simulink model "Wind_Turbine_org"  (Simulink 10.0)
settings: Solver=ode23t  StartTime=0.0  StopTime=70  MaxStep=0.01  RelTol=1e-4  AbsTol=1e-4  EnableMultiTasking=on
PreLoadFcn:
  | warning off Simulink:Commands:LoadMdlParameterizedLink
PostLoadFcn:
  | warning off Simulink:blocks:MatchingGotoNotFound
  | warning off Simulink:blocks:MatchingFromNotFound
  | warning('off','Simulink:SL_OutputNotConnected');
  | warning off Simulink:Engine:SaveWithParameterizedLinks_Warning
  | warning off Simulink:Engine:SaveWithDisabledLinks_Warning
  | warning('off','Simulink:fixpoint:fxpParameterPrecisionLoss');
  | warning off Simulink:blocks:DTConversionUncessary
  | warning off ne_sli:simulator:input:FilteredInputs
  | warning off MATLAB:nearlySingularMatrix
  | 
  | warning off xPCTarget:modeloptions:StackIncrease
  | warning off xPCTarget:sampleTime:sampleTimeInvariance
  | warning off Simulink:blocks:TDelayFixedBuffer
  | 
  | Setup_WT_Configurations
StartFcn:
  | tic
StopFcn:
  | Elapsed_Sim_Time = toc;
  | disp(['Elapsed time is ' num2str(Elapsed_Sim_Time)]);
undefined symbols (not defined in the file): radps2rpm, sigbuilder_block, WT_Params, X, Y, Z
libraries: powerlib x6, sm_lib x6, Wind_Lib x4, Yaw_System_Lib x4, Generator_Lib x3, Pitch_System_Lib x3, Pitch_Controller_Lib x3, Main_Controller_Lib x2, Geartrain_Lib x2, Hub_Axis_Lib x2, Blades_Lib x1, nesl_utility x1
Description:
  | Copyright 2009-2017 The MathWorks, Inc. MathWorks, Inc.
settings Model: Creator=smiller  LastModifiedBy=bhisma  ExtModeTrigDuration=100
settings SolverCC: AutoScaleAbsTol=off  MaxConsecutiveMinStep=5
settings DataIOCC: SaveFinalState=on
settings OptimizationCC: BlockReduction=off  OptimizeBlockIOStorage=off  BufferReuse=off  GlobalBufferReuse=off  ExpressionFolding=off  ExpressionDepthLimit=2147483647  LocalBlockOutputs=off  OptimizeDataStoreBuffers=off  BusAssignmentInplaceUpdate=off
settings DebuggingCC: AlgebraicLoopMsg=error  ArtificialAlgebraicLoopMsg=none  Int32ToFloatConvMsg=none  UnnecessaryDatatypeConvMsg=warning  FcnCallInpInsideContextMsg=warning  AllowSymbolicDim=off  StateNameClashWarn=warning
settings HardwareCC: ProdIntDivRoundTo=Zero  ProdEndianess=LittleEndian  ProdLongLongMode=on  ProdHWDeviceType=Generic->32-bit x86 compatible  TargetBitPerLong=64  TargetBitPerPointer=64  TargetBitPerSizeT=64  TargetBitPerPtrDiffT=64  TargetLongLongMode=on  TargetIntDivRoundTo=Zero  TargetEndianess=LittleEndian  TargetWordSize=64  TargetHWDeviceType=MATLAB Host
settings SFSimCC: SimParseCustomCode=off
settings RTWCC: Description=Simulink Real-Time  SystemTargetFile=slrt.tlc  TemplateMakefile=slrt_default_tmf  RTWCompilerOptimization=on
settings TargetCC: CodeReplacementLibrary=XPC_BLAS  ParMdlRefBuildCompliant=on  ConcurrentExecutionCompliant=on  GeneratePreprocessorConditionals=Use local settings  MatFileLogging=on  PreserveStateflowLocalDataDimensions=off  MATLABClassNameForMDSCustomization=xpcAperiodicCustomization
settings CustomProperty: DataType=string
settings ConfigComp: CovExternalEMLEnable=off  CovSFcnEnable=off
settings SimscapeCC: ExplicitSolverDiagnosticOptions=none  SimscapeNormalizeSystem=off  SimscapeLogType=all  SimscapeLogName=simlog_Wind_Turbine  SimscapeLogLimitData=off
settings SimMechanicsCC: WarnOnRedundantConstraints=off  VisOnUpdateDiagram=on  VisDuringSimulation=on  FramesToBeSkipped=5  AnimationDelay=0  LastVizWinPosition=[16 233 560 424]  CamPosition=[-49.333;156.594;63.1057;]  CamTarget=[-1.98114;98.9678;-2.9194;]  CamUpVector=[0.335262;0.815674;-0.471461;]  CamHeight=16.8988  VisBackgroundColor=[0.678431;0.921569;1;]  DefaultBodyColor=[1;0;0;]
settings ConfigurationSet: Description=SimMechanics 2G
settings ExplorerConfigSet: InternalSimMechanicsExplorerSettings="<ExplorerConfiguration><canonicalview>default</canonicalview><TilePanel><TileInfo><Tiles Columns=\"2\" Count=\"3\" Rows=\"2\"><Column Left=\"2\" Weight=\"0.6616\"/><Column Left=\"1076\" Weight=\"0.3384\"/><Column Left=\"1628\"/><Row Top=\"2\" Weight=\"0.4995\"/><Row Top=\"507\" Weight=\"0.5005\"/><Row Top=\"1014\"/><Tile Height=\"1\" Width=\"1\" X=\"0\" Y=\"0\"/><Tile Height=\"1\" Width=\"1\" X=\"0\" Y=\"1\"/><Tile Height=\"2\" Width=\"1\" X=\"1\" Y=\"0\"/></Tiles></TileInfo><SceneInfo><SceneViewer><BGColor><R>0.80000001192092896</R><G>1</G><B>1</B></BGColor><Camera><Position><X>151.73049973570119</X><Y>118.34405364859263</Y><Z>134.40663706667596</Z></Position><Center><X>-10.795458452286731</X><Y>-8.3649508446642677</Y><Z>101.0263657071233</Z></Center><Up><X>-0.12932527544138767</X><Y>-0.094165770600414006</Y><Z>0.98712095549595125</Z></Up><Left>-10.158594940113018</Left><Right>10.158594940113018</Right><Bottom>-7.1278539082560997</Bottom><Top>7.1278539082560997</Top></Camera></SceneViewer><SceneViewer><BGColor><R>0.80000001192092896</R><G>1</G><B>1</B></BGColor><Camera><Position><X>3.5719318734898633</X><Y>-0.12848459366052295</Y><Z>225.51131574619058</Z></Position><Center><X>-2.4920494569662206</X><Y>-0.0648600322177105</Y><Z>66.260519833710546</Z></Center><Up><X>0.0026243051834802709</X><Y>-0.99999643177881292</Y><Z>-0.00049945164542893202</Z></Up><Left>-11.826399210226041</Left><Right>11.826399210226041</Right><Bottom>-5.4233487502515896</Bottom><Top>5.4233487502515896</Top></Camera></SceneViewer><SceneViewer><BGColor><R>0.80000001192092896</R><G>1</G><B>1</B></BGColor><Camera><Position><X>121.9852231624925</X><Y>91.296071561311123</Y><Z>95.392428744838412</Z></Position><Center><X>2.8343002263369788</X><Y>-1.5967499794196209</Y><Z>70.920706290818515</Z></Center><Up><X>-0.12932527544138767</X><Y>-0.094165770600414006</Y><Z>0.98712095549595125</Z></Up><Left>-36.268603134155278</Left><Right>36.268603134155278</Right><Bottom>-73.406224822998055</Bottom><Top>73.406224822998055</Top></Camera></SceneViewer></SceneInfo></TilePanel></ExplorerConfiguration>"

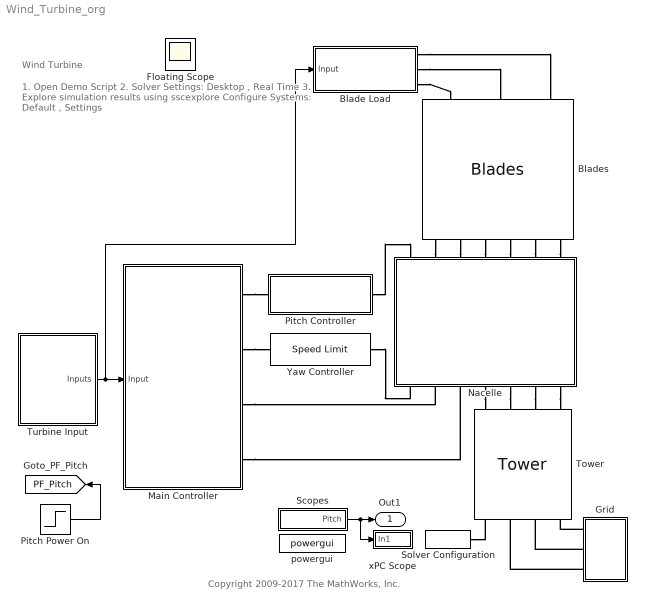
== system Wind_Turbine_org ==
  note: Copyright 2009-2017 The MathWorks, Inc.
  note: 1. Open Demo Script
      | 2. Solver Settings: Desktop , Real Time
      | 3. Explore simulation results using sscexplore
      |
      | Configure Systems: Default , Settings
  note: Wind Turbine
  Blade Load : Subsystem  VariantControlMode=Label  Variant=on  LabelModeActiveChoice=Lift_and_Drag
      settings: AttributesFormatString=%<ActiveVariant>
      mask Display:
      | blk = find_system(gcbh, 'SearchDepth', 1, 'Parent', gcb, 'VariantObject', get_param(gcb,'activevariant'));
      | eval(get_param(blk, 'MaskDisplay'));
  Blades : Blades_Lib/Blades  RequirementInfo={'other' 'wind_turbine_requirements.docx' '@overall_system' 'true' 'Blade Requirements' '' } %GIDa_b4b772d6_2a4e_4d26_8c7e_f4f3f2f69a80  SystemSampleTime=-1
  Grid : Subsystem  RequirementInfo={} %GIDa_31a9dfe5_a537_4323_9f13_a43c2adbc945
  Main Controller : Subsystem  VariantControlMode=Label  Variant=on  LabelModeActiveChoice=Wind_Input
      settings: AttributesFormatString=%<ActiveVariant>
      mask Display:
      | blk = find_system(gcbh, 'SearchDepth', 1, 'Parent', gcb, 'VariantObject', get_param(gcb,'activevariant'));
      | eval(get_param(blk, 'MaskDisplay'));
  Nacelle : Subsystem
      mask Display:
      | PiA_Char = get_param([bdroot '/Nacelle/Pitch System'],'ActiveVariant');
      | YaA_Char = get_param([bdroot '/Nacelle/Yaw System'],'ActiveVariant');
      | Hub_Char = get_param([bdroot '/Nacelle/Hub Axis'],'ActiveVariant');
      | Gea_Char = get_param([bdroot '/Nacelle/Geartrain'],'ActiveVariant');
      | Gen_Char = get_param([bdroot '/Nacelle/Generator'],'ActiveVariant');
      | 
      | if(length(YaA_Char)<7)
      |     YaA_Char = 'LockedL';
      | end
      | 
      | image_str = ['Pi' PiA_Char(1) 'Ya' upper(YaA_Char(7)) 'Hu' Hub_Char(1) 'Ge' Gea_Char(1) 'Gn' Gen_Char(1)];
      | try
      |     image(['Nacelle_' image_str '_IMAGE.jpg']);
      | catch
      |     image('Nacelle_IMAGE.jpg');
      | end
      | 
      | port_label('RConn',1,'YC');
      | port_label('RConn',2,'Br');
      | port_label('RConn',3,'G');
      | port_label('RConn',4,'T');
      | port_label('RConn',5,'GrVa');
      | port_label('RConn',6,'GrVb');
      | port_label('RConn',7,'GrVc');
      | port_label('LConn',1,'PC');
      | port_label('LConn',2,'B1');
      | port_label('LConn',3,'BPA1');
      | port_label('LConn',4,'B2');
      | port_label('LConn',5,'BPA2');
      | port_label('LConn',6,'B3');
      | port_label('LConn',7,'BPA3');
  Pitch Power On : Step  Time=20  Before=24  After=24  SampleTime=0
  Pitch Controller : Subsystem  VariantControlMode=Label  Variant=on  LabelModeActiveChoice=PI_on_AoA
      settings: AttributesFormatString=%<ActiveVariant>
      mask Display:
      | blk = find_system(gcbh, 'SearchDepth', 1, 'Parent', gcb, 'VariantObject', get_param(gcb,'activevariant'));
      | eval(get_param(blk, 'MaskDisplay'));
  Scopes : Subsystem
      mask Display: disp('Scopes');
  Solver Configuration : nesl_utility/Solver Configuration  PhysicalDomain=network_engine_domain  SubClassName=solver  LeftPortType=input  RightPortType=generic  Tones=[]  Harmonics=[]  SimulateNoise=off  Profile=off  UseLocalSampling=off  EnableSwitchedLinearOptims=on  FrequencyDomain=off  UseCCode=off  RelTol=0.001  AbsTol=1e-06  MinStep=1e-09  ToWorkspace=off  RevertToSquareIcSolve=off  NumHomotopyIterations=100  PhasorMode=off  PhasorModeNumHarmonics=1  DoDC=off  ResidualTolerance=1e-9  UseLocalSolver=off  LocalSolverChoice=NE_BACKWARD_EULER_ADVANCER  LocalSolverSampleTime=0.01  DoFixedCost=off  MaxNonlinIter=3  MaxModeIter=2  LinearAlgebra=Sparse  EquationFormulation=NE_TIME_EF  DelaysMemoryBudget=1024  AutomaticFiltering=on  FilteringTimeConstant=0.001  PartitionStorageMethod=AS_NEEDED  PartitionMemoryBudget=1024  PartitionMethod=FAST
  Tower : Tower/Tower  RequirementInfo={} %GIDa_4943b1c2_7ab1_472c_939d_e8be874b5a74  SystemSampleTime=-1
  Turbine Input : Subsystem  VariantControlMode=Label  Variant=on  LabelModeActiveChoice=Wind
      settings: AttributesFormatString=%<ActiveVariant>
      mask Display:
      | blk = find_system(gcbh, 'SearchDepth', 1, 'Parent', gcb, 'VariantObject', get_param(gcb,'activevariant'));
      | eval(get_param(blk, 'MaskDisplay'));
      | 
      | 
      | if strcmp(get_param(gcb,'activevariant'),'Wind')
      |     [gr_ind, l] = signalbuilder([gcb '/Wind/Wind Input'], 'activegroup');
      |     text(0.05,0.9,['Data ' num2str(gr_ind)]);
      | end
  Yaw Controller : Yaw_Controller_Lib/Speed Limit  SystemSampleTime=-1  OverrideUsingVariant=Speed_Limit
  powergui : powerlib/powergui  SimulationMode=Phasor  SampleTime=1e-1  frequency=60  Iterations=50  frequencyindice=60  Pbase=100e6  ErrMax=1e-4  UnitsV=kV  UnitsW=MW  buscounter=0  FunctionMessages=off  echomessages=off  EnableUseOfTLC=off  CurrentSourceSwitches=off  DisableSnubberDevices=off  DisableRonSwitches=off  DisableVfSwitches=off  DisplayEquations=off  AutomaticDiscreteSolvers=off  SolverType=Tustin  Interpol=off  ExternalGateDelay=off  methode=off  Ts=0  x0status=blocks  SPID=off  SwTol=0  HookPort=off  NonlinearTolerance=1e-4  nMaxIteration=100  ContinueOnMaxIteration=off  RestoreLinks=warning  ResistiveCurrentMeasurement=off  Frange=[0:2:500]  Ylog=off  Xlog=on  ShowGrid=off  save=off  variable=ZData  structure=0  ZoomFFT=on  StartTime=0.0  cycles=1  DisplayStyle=1  fundamental=60  FreqAxis=off  MaxFrequency=1000  frequencyindicesteady=1  RmsSteady=1  display=off
      settings: SourceProductName=Simscape Electrical
  xPC Scope : Subsystem
      mask Display: disp('SLRT')
  Out1 : Outport
  Floating Scope : Scope
  tag scope: PF_Pitch=global
  wires:
  Pitch Power On/1 -> [PF_Pitch]
  Turbine Input/1(Inputs) -> Main Controller/1(Input), Blade Load/1(Input)
  Scopes/1(Pitch) -> xPC Scope/1(In1), Out1/1
  connections:
  Blades/LConn1 -- Nacelle/LConn2
  Pitch Controller/RConn1 -- Nacelle/LConn1
  Main Controller/RConn1 -- Pitch Controller/LConn1
  Nacelle/RConn5 -- Tower/LConn2
  Nacelle/RConn4 -- Tower/LConn1
  Solver Configuration/RConn1 -- Tower/RConn1
  Blades/LConn5 -- Nacelle/LConn6
  Blades/LConn4 -- Nacelle/LConn5
  Blades/LConn3 -- Nacelle/LConn4
  Blades/LConn2 -- Nacelle/LConn3
  Blades/LConn6 -- Nacelle/LConn7
  Nacelle/RConn6 -- Tower/LConn3
  Nacelle/RConn7 -- Tower/LConn4
  Grid/RConn1 -- Tower/RConn4
  Grid/RConn2 -- Tower/RConn3
  Grid/RConn3 -- Tower/RConn2
  Main Controller/RConn2 -- Yaw Controller/LConn1
  Main Controller/RConn4 -- Nacelle/RConn3
  Main Controller/RConn3 -- Nacelle/RConn2
  Blade Load/RConn3 -- Blades/RConn1
  Blade Load/RConn2 -- Blades/RConn2
  Blade Load/RConn1 -- Blades/RConn3
  Yaw Controller/RConn1 -- Nacelle/RConn1

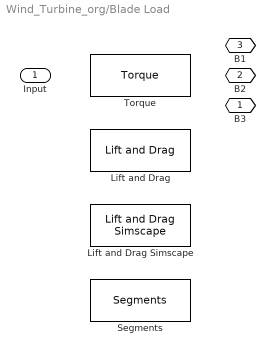
== system Wind_Turbine_org/Blade Load ==
  Input : Inport
  Lift and Drag : Wind_Lib/Lift and Drag  SystemSampleTime=-1  VariantControl=Lift_and_Drag
  Lift and Drag Simscape : Wind_Lib/Lift and Drag Simscape  SystemSampleTime=-1  VariantControl=Lift_and_Drag_Simscape
  Segments : Wind_Lib/Segments  SystemSampleTime=-1  VariantControl=Segments
  Torque : Wind_Lib/Torque  SystemSampleTime=-1  VariantControl=Torque
  B3 : PMIOPort  Side=Right
  B2 : PMIOPort  Port=2  Side=Right
  B1 : PMIOPort  Port=3  Side=Right

== system Wind_Turbine_org/Grid ==
  note: Copyright 2009-2017 The MathWorks, Inc.
  "1 km line " : powerlib/Elements/Three-Phase PI Section Line  LConnTagsString=a|b|c  RConnTagsString=A|B|C  Frequency=WT_Params.Grid.frequency  Resistances=[0.1153 0.413]  Inductances=[1.05e-3 3.32e-3]  Capacitances=[11.33e-009 5.01e-009]  Length=1
      settings: SourceProductName=Simscape Electrical
  Grid : powerlib/Electrical Sources/Three-Phase Programmable Voltage Source  PositiveSequence=[WT_Params.Grid.voltage 0 WT_Params.Grid.frequency]  VariationEntity=None  VariationType=Table of time-amplitude pairs  VariationTypeAlt=Step  VariationStep=-0.15  VariationRate=10  VariationMagnitude=0.3  VariationFrequency=2  VariationTiming=[5 5.5]  VariationPhaseA=off  Amplitudes="[1.0  0.5  1.0 ]"  TimeValues="[0  10  10.1]"  HarmonicGeneration=off  HarmonicA=[1 -0.1 0 1]  HarmonicB=[2 0.15 35 2]  Timing="[5  5.5]"  BusType=swing  Pref=0  Qref=0  Qmin=-inf  Qmax=inf
      settings: SourceProductName=Simscape Electrical
  Ground1 : powerlib/Elements/Ground  LConnTagsString=a
      settings: SourceProductName=Simscape Electrical
  Line Resistance : powerlib/Elements/Three-Phase Mutual Inductance Z1-Z0  LConnTagsString=a|b|c  RConnTagsString=A|B|C  PositiveSequence="[0.1  1.0/(2*pi*60)]*WT_Params.Grid.voltage^2/2500e6"  ZeroSequence="[0.3  3.0/(2*pi*60)]*WT_Params.Grid.voltage^2/2500e6"
      settings: SourceProductName=Simscape Electrical  SourceProductBaseCode=PS
  mGrid : powerlib/Measurements/Three-Phase V-I Measurement  VoltageMeasurement=phase-to-ground  SetLabelV=on  LabelV=VmGrid  Vpu=on  VpuLL=off  CurrentMeasurement=no  SetLabelI=on  LabelI=ImGrid  Ipu=off  Pbase=1.5e6/0.9  Vbase=25e3  OutputType=Magnitude  PhasorSimulation=on  PSBequivalent=0
      settings: SourceProductName=Simscape Electrical
  GNVc : PMIOPort  Side=Right
  GNVb : PMIOPort  Port=2  Side=Right
  GNVa : PMIOPort  Port=3  Side=Right
  connections:
  Line Resistance/RConn1 -- "1 km line "/LConn1
  "1 km line "/LConn2 -- Line Resistance/RConn2
  Line Resistance/RConn3 -- "1 km line "/LConn3
  Grid/LConn1 -- Ground1/LConn1
  Grid/RConn1 -- mGrid/LConn1
  mGrid/LConn2 -- Grid/RConn2
  Grid/RConn3 -- mGrid/LConn3
  mGrid/RConn1 -- Line Resistance/LConn1
  Line Resistance/LConn2 -- mGrid/RConn2
  mGrid/RConn3 -- Line Resistance/LConn3
  GNVa/RConn1 -- "1 km line "/RConn1
  GNVb/RConn1 -- "1 km line "/RConn2
  GNVc/RConn1 -- "1 km line "/RConn3

== system Wind_Turbine_org/Main Controller ==
  Input : Inport
  Direct Input : Main_Controller_Lib/Direct Input  SystemSampleTime=-1  VariantControl=Direct_Input
  Wind Input : Main_Controller_Lib/Wind Input  SystemSampleTime=-1  VariantControl=Wind_Input
  PC : PMIOPort  Tag=PMCPort  Side=Right
  YC : PMIOPort  Tag=PMCPort  Port=2  Side=Right
  Br : PMIOPort  Tag=PMCPort  Port=3  Side=Right
  G : PMIOPort  Tag=PMCPort  Port=4  Side=Right

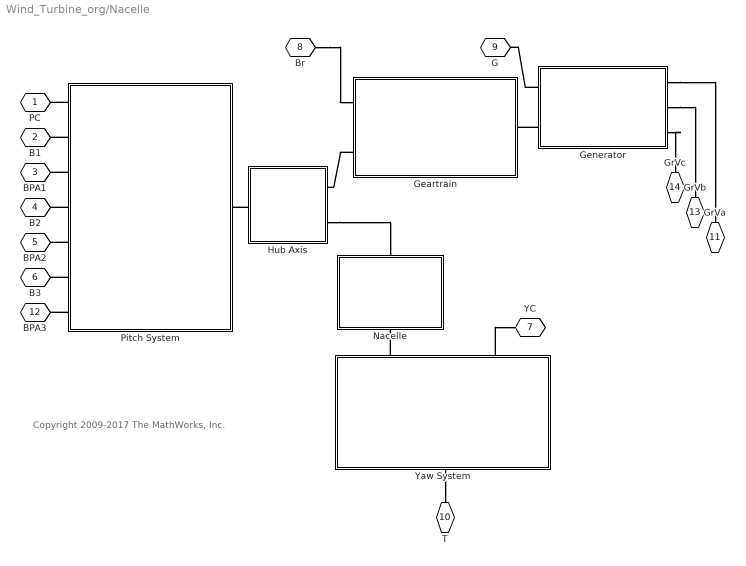
== system Wind_Turbine_org/Nacelle ==
  note: Copyright 2009-2017 The MathWorks, Inc.
  Geartrain : Subsystem  RequirementInfo={'other' 'Wind_Turbine_Requirements.docx' '@Simulink_requirement_item_4' 'true' 'Geartrain Requirements' '' } %GIDa_0de6bbf9_bd2a_4f23_951e_791819310b87  VariantControlMode=Label  Variant=on  LabelModeActiveChoice=Ideal
      settings: AttributesFormatString=%<ActiveVariant>
      mask Display:
      | blk = find_system(gcbh, 'SearchDepth', 1, 'Parent', gcb, 'VariantObject', get_param(gcb,'activevariant'));
      | eval(get_param(blk, 'MaskDisplay'));
  Generator : Subsystem  RequirementInfo={'other' 'Wind_Turbine_Requirements.docx' '@Simulink_requirement_item_5' 'true' 'Generator Requirements' '' } %GIDa_fc3d0265_e5fe_47b9_917a_323d12640d23  VariantControlMode=Label  Variant=on  LabelModeActiveChoice=Full
      settings: AttributesFormatString=%<ActiveVariant>
      mask Display:
      | blk = find_system(gcbh, 'SearchDepth', 1, 'Parent', gcb, 'VariantObject', get_param(gcb,'activevariant'));
      | eval(get_param(blk, 'MaskDisplay'));
  Hub Axis : Subsystem  Tag=CustomStyle  VariantControlMode=Label  Variant=on  LabelModeActiveChoice=Rotate
      settings: AttributesFormatString=%<ActiveVariant>
      mask Display:
      | blk = find_system(gcbh, 'SearchDepth', 1, 'Parent', gcb, 'VariantObject', get_param(gcb,'activevariant'));
      | eval(get_param(blk, 'MaskDisplay'));
  Nacelle : Subsystem
      mask Display:
      | image('Nacelle_Housing_IMAGE.jpg');
      | port_label('RConn',1,'N');
      | port_label('LConn',1,'YR');
  Pitch System : Subsystem  Tag=CustomStyle  VariantControlMode=Label  Variant=on  LabelModeActiveChoice=Ideal
      settings: AttributesFormatString=%<ActiveVariant>
      mask Display:
      | blk = find_system(gcbh, 'SearchDepth', 1, 'Parent', gcb, 'VariantObject', get_param(gcb,'activevariant'));
      | eval(get_param(blk, 'MaskDisplay'));
  Yaw System : Subsystem  Tag=CustomStyle  VariantControlMode=Label  Variant=on  LabelModeActiveChoice=Ideal_Actuator
      settings: AttributesFormatString=%<ActiveVariant>
      mask Display:
      | blk = find_system(gcbh, 'SearchDepth', 1, 'Parent', gcb, 'VariantObject', get_param(gcb,'activevariant'));
      | eval(get_param(blk, 'MaskDisplay'));
  PC : PMIOPort  Tag=PMCPort  Side=Left
  B1 : PMIOPort  Tag=PMCPort  Port=2  Side=Left
  BPA1 : PMIOPort  Tag=PMCPort  Port=3  Side=Left
  B2 : PMIOPort  Tag=PMCPort  Port=4  Side=Left
  BPA2 : PMIOPort  Tag=PMCPort  Port=5  Side=Left
  B3 : PMIOPort  Tag=PMCPort  Port=6  Side=Left
  YC : PMIOPort  Tag=PMCPort  Port=7  Side=Right
  Br : PMIOPort  Tag=PMCPort  Port=8  Side=Right
  G : PMIOPort  Tag=PMCPort  Port=9  Side=Right
  T : PMIOPort  Tag=PMCPort  Port=10  Side=Right
  GrVa : PMIOPort  Tag=PMCPort  Port=11  Side=Right
  BPA3 : PMIOPort  Tag=PMCPort  Port=12  Side=Left
  GrVb : PMIOPort  Tag=PMCPort  Port=13  Side=Right
  GrVc : PMIOPort  Tag=PMCPort  Port=14  Side=Right
  connections:
  Hub Axis/LConn1 -- Pitch System/RConn1
  Yaw System/RConn1 -- Nacelle/LConn1
  Yaw System/LConn1 -- T/RConn1
  Generator/RConn3 -- GrVc/RConn1
  Generator/RConn2 -- GrVb/RConn1
  Br/RConn1 -- Geartrain/LConn1
  Pitch System/LConn7 -- BPA3/RConn1
  Pitch System/LConn5 -- BPA2/RConn1
  Pitch System/LConn3 -- BPA1/RConn1
  Pitch System/LConn6 -- B3/RConn1
  Generator/LConn2 -- Geartrain/RConn1
  Generator/LConn1 -- G/RConn1
  Generator/RConn1 -- GrVa/RConn1
  Pitch System/LConn1 -- PC/RConn1
  Pitch System/LConn4 -- B2/RConn1
  Pitch System/LConn2 -- B1/RConn1
  Hub Axis/RConn2 -- Nacelle/RConn1
  Yaw System/RConn2 -- YC/RConn1
  Geartrain/LConn2 -- Hub Axis/RConn1

== system Wind_Turbine_org/Pitch Controller ==
  Inner Loop : Pitch_Controller_Lib/Inner Loop  SystemSampleTime=-1  VariantControl=Inner_Loop
  PI on AoA : Pitch_Controller_Lib/PI on AoA  SystemSampleTime=-1  VariantControl=PI_on_AoA
  PI on AoA Code : Pitch_Controller_Lib/PI on AoA Code  SystemSampleTime=-1  VariantControl=PI_on_AoA_Code
  P : PMIOPort  Tag=PMCPort  Side=Right
  M : PMIOPort  Tag=PMCPort  Port=2  Side=Left

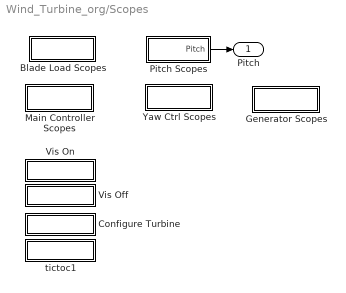
== system Wind_Turbine_org/Scopes ==
  Blade Load Scopes : Subsystem  AncestorBlock=Wind_Lib/Blade Load Scopes
  Configure Turbine : Subsystem
      mask Display: disp('Configs');
  Generator Scopes : Subsystem  AncestorBlock=Generator_Lib/Generator Scopes
  Main Controller Scopes : Subsystem  AncestorBlock=Main_Controller_Lib/Main Controller Scopes
  Pitch Scopes : Subsystem  AncestorBlock=Pitch_Controller_Lib/Pitch Scopes
  Vis Off : Subsystem
      settings: OpenFcn=set_param(bdroot,'SimMechanicsOpenEditorOnUpdate','off');
      mask Display: disp('Vis Off')
  Vis On : Subsystem
      settings: OpenFcn=set_param(bdroot,'SimMechanicsOpenEditorOnUpdate','on');
      mask Display: disp('Vis On')
  Yaw Ctrl Scopes : Subsystem  AncestorBlock=Yaw_Controller_Lib/Yaw Ctrl Scopes
  tictoc1 : Subsystem
      settings: OpenFcn=open('Wind_Turbine_Demo_Script.html')
      mask Display: disp('Script')
  Pitch : Outport
  wires:
  Pitch Scopes/1(Pitch) -> Pitch/1

== system Wind_Turbine_org/Turbine Input ==
  Commands : Subsystem  VariantControl=Commands
      mask Display:
      | image(imread('Turbine_Input_Commands_IMAGE.jpg'));
      | port_label('output',1,'Inputs');
  Wind : Subsystem  VariantControl=Wind
      mask Display:
      | image('Turbine_Input_Wind_IMAGE.jpg');
      | port_label('output',1,'Inputs');
  Inputs : Outport

== system Wind_Turbine_org/xPC Scope ==
  In1 : Inport
  "Scope (SLRT) " : slrtlib/Displays and Logging/Scope   scopeno=1  scopetype=Target  autostart=on  viewmode=Graphical redraw  formatstr='%15.6f'  grid=on  ylimits=[-5 70]  nosamples=200  noprepostsamples=0  interleave=1  triggermode=FreeRun  triggersignal=1  trigsignalfromport=off  triggerlevel=0.0  triggerslope=Either  triggerscope=1  triggersample=0  filename=data.dat  mode=Lazy  writesize=512  autorestart=off  dynamicfilemode=off  maxwritefilesize=512*1024^2
  wires:
  In1/1 -> "Scope (SLRT) "/1

== system Wind_Turbine_org/Nacelle/Geartrain ==
  Empty : Geartrain_Lib/Empty  SystemSampleTime=-1  VariantControl=Empty
  Ideal : Geartrain_Lib/Ideal  SystemSampleTime=-1  VariantControl=Ideal
  BC : PMIOPort  Tag=PMCPort  Side=Left
  R : PMIOPort  Tag=PMCPort  Port=2  Side=Left
  GN : PMIOPort  Tag=PMCPort  Port=3  Side=Right

== system Wind_Turbine_org/Nacelle/Generator ==
  Full : Generator_Lib/Full  SystemSampleTime=-1  VariantControl=Full
  Simple : Generator_Lib/Simple  SystemSampleTime=-1  VariantControl=Simple
  M : PMIOPort  Tag=PMCPort  Side=Left
  G : PMIOPort  Port=2  Side=Left
  GrVa : PMIOPort  Port=3  Side=Right
  GrVb : PMIOPort  Port=4  Side=Right
  GrVc : PMIOPort  Port=5  Side=Right

== system Wind_Turbine_org/Nacelle/Hub Axis ==
  Locked : Hub_Axis_Lib/Locked  SystemSampleTime=-1  VariantControl=Locked
  Rotate : Hub_Axis_Lib/Rotate  SystemSampleTime=-1  VariantControl=Rotate
  G : PMIOPort  Side=Right
  R : PMIOPort  Port=2  Side=Left
  N : PMIOPort  Port=3  Side=Right

== system Wind_Turbine_org/Nacelle/Nacelle ==
  Geometry : sm_lib/Body Elements/Extruded Solid  GraphicAmbientColor=[0.15 0.15 0.15 1.0]  BasedOnType=Density  CenterOfMass=[0 0 0]  CenterOfMassUnits=m  GraphicDiffuseColor=[0.8 0.8 0.8]  ExtrusionCrossSection=WT_Params.Nacelle.Geometry.profile  ExtrusionCrossSectionUnits=m  Density=1000  DensityUnits=kg/(m^3)  DoExposeReferenceFrame=on  GraphicEmissiveColor=[0.0 0.0 0.0 1.0]  ExportEntireGeometry=off  ExtrusionLength=WT_Params.Nacelle.length  ExtrusionLengthUnits=m  ExtrusionType=General  SerializedFrames=<Frames/>  MarkerShape=Sphere  MarkerSize=10  GraphicType=FromGeometry  InertiaType=PointMass  Mass=0.1  MassUnits=kg  MomentsOfInertia=[1 1 1]  MomentsOfInertiaUnits=kg*m^2  PolygonNumSides=3  GraphicOpacity=1.0  PolygonOuterRadius=1  PolygonOuterRadiusUnits=m  ProductsOfInertia=[0 0 0]  ProductsOfInertiaUnits=kg*m^2  GraphicShininess=75  GraphicSpecularColor=[0.5 0.5 0.5 1.0]  GraphicVisPropType=SimpleVisualProperties
      settings: SourceProductName=Simscape Multibody
  Inertia : sm_lib/Body Elements/Spherical Solid  GraphicAmbientColor=[0.15 0.15 0.15 1.0]  BasedOnType=Density  CenterOfMass=[0 0 0]  CenterOfMassUnits=m  GraphicDiffuseColor=[0.8 0.8 0.8]  Density=1000  DensityUnits=kg/(m^3)  DoExposeReferenceFrame=on  GraphicEmissiveColor=[0.0 0.0 0.0 1.0]  ExportEntireGeometry=off  SerializedExposedGeometries=<ExposedGeometries/>  SerializedFrames=<Frames/>  MarkerShape=Sphere  MarkerSize=10  GraphicType=FromGeometry  InertiaType=Custom  Mass=WT_Params.Nacelle.mass  MassUnits=kg  MomentsOfInertia=[WT_Params.Nacelle.inertia(1,1) WT_Params.Nacelle.inertia(3,3) WT_Params.Nacelle.inertia(2,2)]  MomentsOfInertiaUnits=kg*m^2  GraphicOpacity=1.0  ProductsOfInertia=[0 0 0]  ProductsOfInertiaUnits=kg*m^2  GraphicShininess=75  GraphicSpecularColor=[0.5 0.5 0.5 1.0]  SphereRadius=0.1  SphereRadiusUnits=m  GraphicVisPropType=SimpleVisualProperties
      settings: SourceProductName=Simscape Multibody
  Transform Extrusion : sm_lib/Frames and Transforms/Rigid Transform  TranslationMethod=Cartesian  TranslationStandardOffset=1  TranslationLengthUnit=m  TranslationStandardAxis=+Z  TranslationCartesianOffset=[0 0 0]  TranslationROffset=0  TranslationROffsetUnits=m  TranslationZOffset=0  TranslationZOffsetUnits=m  TranslationThetaOffset=0  TranslationThetaOffsetUnits=deg  RotationMethod=StandardAxis  RotationAngleUnits=deg  RotationStandardAxis=+Y  RotationAngle=90  RotationArbitraryAxis=[0 0 1]  FollAlignAxisA=+X  BaseAlignAxisA=+Y  FollAlignAxisB=+Y  BaseAlignAxisB=+Z  RotationSequenceAxes=FollowerAxes  RotationSequence=XYX  RotationSequenceAngles=[0 0 0]  RotationSequenceAnglesUnits=deg  RotationMatrix=[1 0 0; 0 1 0; 0 0 1]
  Transform Hub Center : sm_lib/Frames and Transforms/Rigid Transform  TranslationMethod=StandardAxis  TranslationStandardOffset=WT_Params.Nacelle.length/2  TranslationLengthUnit=m  TranslationStandardAxis=+X  TranslationCartesianOffset=[0 0 0]  TranslationROffset=0  TranslationROffsetUnits=m  TranslationZOffset=0  TranslationZOffsetUnits=m  TranslationThetaOffset=0  TranslationThetaOffsetUnits=deg  RotationMethod=StandardAxis  RotationAngleUnits=deg  RotationStandardAxis=+Y  RotationAngle=90  RotationArbitraryAxis=[0 0 1]  FollAlignAxisA=+X  BaseAlignAxisA=+Y  FollAlignAxisB=+Y  BaseAlignAxisB=+Z  RotationSequenceAxes=FollowerAxes  RotationSequence=XYX  RotationSequenceAngles=[0 0 0]  RotationSequenceAnglesUnits=deg  RotationMatrix=[1 0 0; 0 1 0; 0 0 1]
  Transform Nacelle CG : sm_lib/Frames and Transforms/Rigid Transform  TranslationMethod=Cartesian  TranslationStandardOffset=1  TranslationLengthUnit=m  TranslationStandardAxis=+Z  TranslationCartesianOffset=[-WT_Params.Nacelle.Yaw_Ctr_Offset.x+WT_Params.Nacelle.CG_Offset.x 0 WT_Params.Nacelle.Yaw_Ctr_Offset.y]  TranslationROffset=0  TranslationROffsetUnits=m  TranslationZOffset=0  TranslationZOffsetUnits=m  TranslationThetaOffset=0  TranslationThetaOffsetUnits=deg  RotationMethod=None  RotationAngleUnits=deg  RotationStandardAxis=+Z  RotationAngle=0  RotationArbitraryAxis=[0 0 1]  FollAlignAxisA=+X  BaseAlignAxisA=+Y  FollAlignAxisB=+Y  BaseAlignAxisB=+Z  RotationSequenceAxes=FollowerAxes  RotationSequence=XYX  RotationSequenceAngles=[0 0 0]  RotationSequenceAnglesUnits=deg  RotationMatrix=[1 0 0; 0 1 0; 0 0 1]
  Transform Nacelle Ctr : sm_lib/Frames and Transforms/Rigid Transform  TranslationMethod=Cartesian  TranslationStandardOffset=1  TranslationLengthUnit=m  TranslationStandardAxis=+Z  TranslationCartesianOffset=[-WT_Params.Nacelle.length/2+3 0 WT_Params.Nacelle.Yaw_Ctr_Offset.y]  TranslationROffset=0  TranslationROffsetUnits=m  TranslationZOffset=0  TranslationZOffsetUnits=m  TranslationThetaOffset=0  TranslationThetaOffsetUnits=deg  RotationMethod=None  RotationAngleUnits=deg  RotationStandardAxis=+Z  RotationAngle=0  RotationArbitraryAxis=[0 0 1]  FollAlignAxisA=+X  BaseAlignAxisA=+Y  FollAlignAxisB=+Y  BaseAlignAxisB=+Z  RotationSequenceAxes=FollowerAxes  RotationSequence=XYX  RotationSequenceAngles=[0 0 0]  RotationSequenceAnglesUnits=deg  RotationMatrix=[1 0 0; 0 1 0; 0 0 1]
  N : PMIOPort  Side=Right
  YR : PMIOPort  Port=2  Side=Left
  connections:
  Transform Nacelle Ctr/LConn1 -- YR/RConn1 -- Transform Nacelle CG/LConn1
  Transform Nacelle Ctr/RConn1 -- Transform Extrusion/LConn1 -- Transform Hub Center/LConn1
  Transform Hub Center/RConn1 -- N/RConn1
  Inertia/RConn1 -- Transform Nacelle CG/RConn1
  Transform Extrusion/RConn1 -- Geometry/RConn1

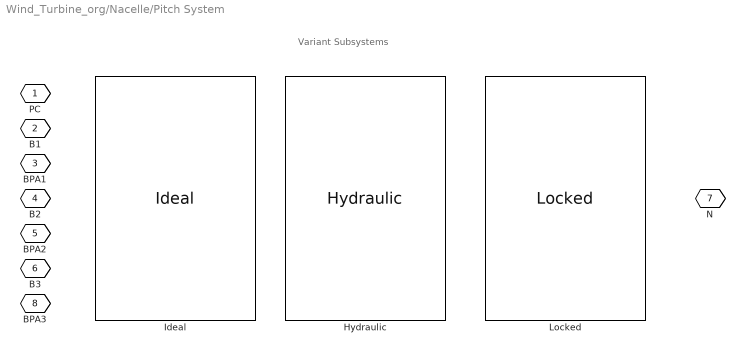
== system Wind_Turbine_org/Nacelle/Pitch System ==
  note: Variant Subsystems
  Hydraulic : Pitch_System_Lib/Hydraulic  SystemSampleTime=-1  VariantControl=Hydraulic
  Ideal : Pitch_System_Lib/Ideal  SystemSampleTime=-1  VariantControl=Ideal
  Locked : Pitch_System_Lib/Locked  SystemSampleTime=-1  VariantControl=Locked
  PC : PMIOPort  Tag=PMCPort  Side=Left
  B1 : PMIOPort  Tag=PMCPort  Port=2  Side=Left
  BPA1 : PMIOPort  Tag=PMCPort  Port=3  Side=Left
  B2 : PMIOPort  Tag=PMCPort  Port=4  Side=Left
  BPA2 : PMIOPort  Tag=PMCPort  Port=5  Side=Left
  B3 : PMIOPort  Tag=PMCPort  Port=6  Side=Left
  N : PMIOPort  Tag=PMCPort  Port=7  Side=Right
  BPA3 : PMIOPort  Tag=PMCPort  Port=8  Side=Left

== system Wind_Turbine_org/Nacelle/Yaw System ==
  Ideal Actuator : Yaw_System_Lib/Ideal Actuator  SystemSampleTime=-1  VariantControl=Ideal_Actuator
  Ideal Motor : Yaw_System_Lib/Ideal Motor  SystemSampleTime=-1  VariantControl=Ideal_Motor
  Locked : Yaw_System_Lib/Locked  SystemSampleTime=-1  VariantControl=Locked
  Servomotor : Yaw_System_Lib/Servomotor  SystemSampleTime=-1  VariantControl=Servomotor
  N : PMIOPort  Side=Right
  T : PMIOPort  Port=2  Side=Left
  YC : PMIOPort  Port=3  Side=Right

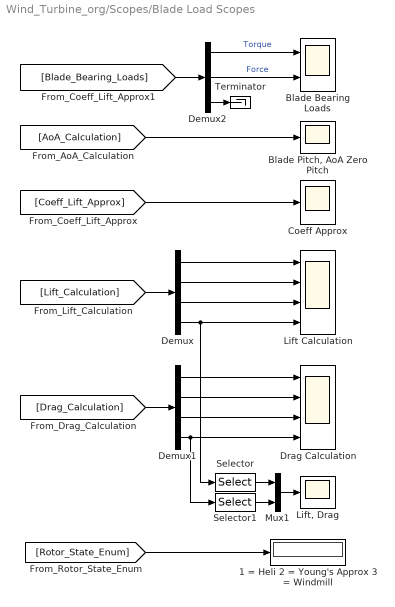
== system Wind_Turbine_org/Scopes/Blade Load Scopes ==
  1 = Heli 2 = Young's Approx 3 = Windmill : Display
  Blade Bearing Loads : Scope  NumInputPorts=2
  "Blade Pitch, AoA Zero Pitch" : Scope
  Coeff Approx : Scope
  Demux : Demux  Outputs=[1 3 3 3]
  Demux1 : Demux  Outputs=[1 3 3 3]
  Demux2 : Demux  Outputs=[3 3 12]
  Drag Calculation : Scope  NumInputPorts=4
  Lift Calculation : Scope  NumInputPorts=4
  "Lift, Drag" : Scope
  Mux1 : Mux  Inputs=2
  Selector : Selector  InputPortWidth=3  IndexOptions=Index vector (dialog)  Indices=[1]  OutputSizes=1
  Selector1 : Selector  InputPortWidth=3  IndexOptions=Index vector (dialog)  Indices=[1 3]  OutputSizes=1
  Terminator : Terminator
  wires:
  Demux2/3 -> Terminator/1
  [Rotor_State_Enum] -> 1 = Heli 2 = Young's Approx 3 = Windmill/1
  Demux1/4 -> Drag Calculation/4, Selector1/1
  Demux1/3 -> Drag Calculation/3
  Demux1/2 -> Drag Calculation/2
  Demux1/1 -> Drag Calculation/1
  [Drag_Calculation] -> Demux1/1
  [Coeff_Lift_Approx] -> Coeff Approx/1
  Demux/4 -> Lift Calculation/4, Selector/1
  Demux/3 -> Lift Calculation/3
  Demux/2 -> Lift Calculation/2
  Demux/1 -> Lift Calculation/1
  [Lift_Calculation] -> Demux/1
  Mux1/1 -> "Lift, Drag"/1
  [AoA_Calculation] -> "Blade Pitch, AoA Zero Pitch"/1
  Selector/1 -> Mux1/1
  Selector1/1 -> Mux1/2
  [Blade_Bearing_Loads] -> Demux2/1
  Demux2/1 -> Blade Bearing Loads/1  "Torque"
  Demux2/2 -> Blade Bearing Loads/2  "Force"

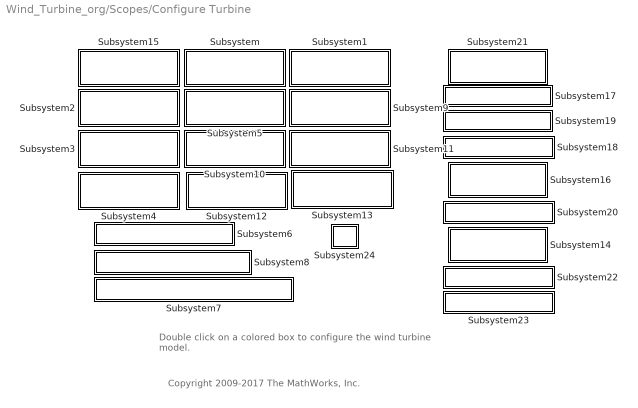
== system Wind_Turbine_org/Scopes/Configure Turbine ==
  note: Copyright 2009-2017 The MathWorks, Inc.
  note: Double click on a colored box
      | to configure the wind turbine model.
  Subsystem : Subsystem
      settings: OpenFcn=Select_Turbine_Systems('I_Pitch Test', WT_Configs)
      mask Display: disp('Ideal\nPitch')
  Subsystem1 : Subsystem
      settings: OpenFcn=Select_Turbine_Systems('H_Pitch Test', WT_Configs)
      mask Display: disp('Hydraulic\nPitch')
  Subsystem10 : Subsystem
      settings: OpenFcn=Select_Turbine_Systems('I_Pitch IM_Yaw Test', WT_Configs)
      mask Display: disp('Ideal Pitch\nIdeal Motor Yaw')
  Subsystem11 : Subsystem
      settings: OpenFcn=Select_Turbine_Systems('H_Pitch IM_Yaw Test', WT_Configs)
      mask Display: disp('Hydraulic Pitch\nIdeal Motor Yaw')
  Subsystem12 : Subsystem
      settings: OpenFcn=Select_Turbine_Systems('I_Pitch S_Yaw Test', WT_Configs)
      mask Display: disp('Ideal Pitch\nServomotor Yaw')
  Subsystem13 : Subsystem
      settings: OpenFcn=Select_Turbine_Systems('H_Pitch S_Yaw Test', WT_Configs)
      mask Display: disp('Hydraulic Pitch\nServomotor Yaw')
  Subsystem14 : Subsystem
      settings: OpenFcn=Compare_Yaw_Actuators;
      mask Display: disp('Compare Yaw\nActuators')
  Subsystem15 : Subsystem
      mask Display: disp('TESTS')
  Subsystem16 : Subsystem
      settings: OpenFcn=Compare_Pitch_Actuators;
      mask Display: disp('Compare Pitch\nActuators')
  Subsystem17 : Subsystem
      settings: OpenFcn=Pitch_Actuation_Linkage
      mask Display: disp('Pitch Linkage')
  Subsystem18 : Subsystem
      settings: OpenFcn=Pitch_Actuation_Hydraulic_Testrig
      mask Display: disp('Hydr. Pitch Testrig')
  Subsystem19 : Subsystem
      settings: OpenFcn=Pitch_Control_Ideal_Testrig
      mask Display: disp('Ideal Pitch Testrig')
  Subsystem2 : Subsystem
      settings: OpenFcn=Select_Turbine_Systems('IA_Yaw Test', WT_Configs)
      mask Display: disp('Ideal Actuator\nYaw')
  Subsystem20 : Subsystem
      settings: OpenFcn=Yaw_Actuation_Testrig
      mask Display: disp('Yaw Testrig')
  Subsystem21 : Subsystem
      mask Display: disp('DEVELOP')
  Subsystem22 : Subsystem
      settings: OpenFcn=Generator_Testrig
      mask Display: disp('Generator Testrig')
  Subsystem23 : Subsystem
      settings: OpenFcn=Turbine_State_Machine_Testrig
      mask Display: disp('Supervisory Ctrl')
  Subsystem24 : Subsystem
      settings: OpenFcn=Select_Turbine_Systems('H_Pitch S_Yaw Ge Gn Lift_Drag', WT_Configs)
      mask Display: disp('C')
  Subsystem3 : Subsystem
      settings: OpenFcn=Select_Turbine_Systems('IM_Yaw Test', WT_Configs)
      mask Display: disp('Ideal Motor\nYaw')
  Subsystem4 : Subsystem
      settings: OpenFcn=Select_Turbine_Systems('S_Yaw Test', WT_Configs)
      mask Display: disp('Servomotor\nYaw')
  Subsystem5 : Subsystem
      settings: OpenFcn=Select_Turbine_Systems('I_Pitch IA_Yaw Test', WT_Configs)
      mask Display: disp('Ideal Pitch\nIdeal Act. Yaw')
  Subsystem6 : Subsystem
      settings: OpenFcn=Select_Turbine_Systems('I_Pitch IA_Yaw Lift_Drag', WT_Configs)
      mask Display: disp('I Pitch IA Yaw Lift Drag')
  Subsystem7 : Subsystem
      settings: OpenFcn=Select_Turbine_Systems('I_Pitch IA_Yaw Ge Gn Lift_Drag', WT_Configs)
      mask Display: disp('I_Pitch IA_Yaw Ge Gn Lift_Drag')
  Subsystem8 : Subsystem
      settings: OpenFcn=Select_Turbine_Systems('I_Pitch IA_Yaw Ge Lift_Drag', WT_Configs)
      mask Display: disp('I Pitch IA Yaw Ge Lift Drag')
  Subsystem9 : Subsystem
      settings: OpenFcn=Select_Turbine_Systems('H_Pitch IA_Yaw Test', WT_Configs)
      mask Display: disp('Hydraulic Pitch\nIdeal Act. Yaw')

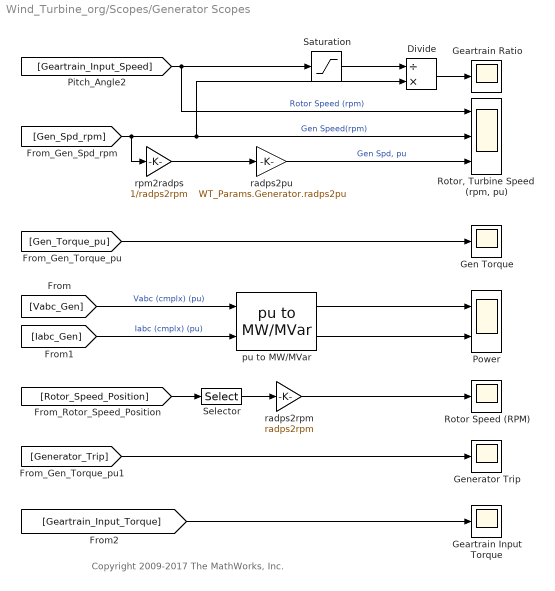
== system Wind_Turbine_org/Scopes/Generator Scopes ==
  note: Copyright 2009-2017 The MathWorks, Inc.
  Divide : Product  Inputs=/*
  Geartrain Input Torque : Scope
  Geartrain Ratio : Scope
  Gen Torque : Scope
  Generator Trip : Scope
  Power : Scope  NumInputPorts=2
  Rotor Speed (RPM) : Scope
  "Rotor, Turbine Speed  (rpm, pu)" : Scope  NumInputPorts=3
  Saturation : Saturate  UpperLimit=inf  LowerLimit=eps
  Selector : Selector  InputPortWidth=2  IndexOptions=Index vector (dialog)  Indices=[2]  OutputSizes=1
  pu to MW/MVar : Generator_Lib/Generator Scopes/pu to MW//MVar
  radps2pu : Gain  Gain=WT_Params.Generator.radps2pu
  radps2rpm : Gain  Gain=radps2rpm
  rpm2radps : Gain  Gain=1/radps2rpm
  wires:
  [Generator_Trip] -> Generator Trip/1
  pu to MW/MVar/2 -> Power/2
  pu to MW/MVar/1 -> Power/1
  [Gen_Torque_pu] -> Gen Torque/1
  [Iabc_Gen] -> pu to MW/MVar/2  "Iabc (cmplx) (pu)"
  [Vabc_Gen] -> pu to MW/MVar/1  "Vabc (cmplx) (pu)"
  [Geartrain_Input_Speed] -> "Rotor, Turbine Speed  (rpm, pu)"/1, Saturation/1  "Rotor Speed (rpm)"
  radps2pu/1 -> "Rotor, Turbine Speed  (rpm, pu)"/3  "Gen Spd, pu"
  rpm2radps/1 -> radps2pu/1
  Divide/1 -> Geartrain Ratio/1
  [Gen_Spd_rpm] -> "Rotor, Turbine Speed  (rpm, pu)"/2, Divide/2, rpm2radps/1  "Gen Speed(rpm)"
  [Rotor_Speed_Position] -> Selector/1
  Selector/1 -> radps2rpm/1
  radps2rpm/1 -> Rotor Speed (RPM)/1
  Saturation/1 -> Divide/1
  [Geartrain_Input_Torque] -> Geartrain Input Torque/1

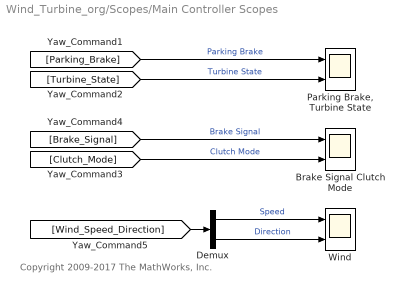
== system Wind_Turbine_org/Scopes/Main Controller Scopes ==
  note: Copyright 2009-2017 The MathWorks, Inc.
  Brake Signal Clutch Mode : Scope  NumInputPorts=2
  Demux : Demux  Outputs=2
  "Parking Brake, Turbine State" : Scope  NumInputPorts=2
  Wind : Scope  NumInputPorts=2
  wires:
  [Parking_Brake] -> "Parking Brake, Turbine State"/1  "Parking Brake"
  [Turbine_State] -> "Parking Brake, Turbine State"/2  "Turbine State"
  [Brake_Signal] -> Brake Signal Clutch Mode/1  "Brake Signal"
  [Clutch_Mode] -> Brake Signal Clutch Mode/2  "Clutch Mode"
  [Wind_Speed_Direction] -> Demux/1
  Demux/1 -> Wind/1  "Speed"
  Demux/2 -> Wind/2  "Direction"

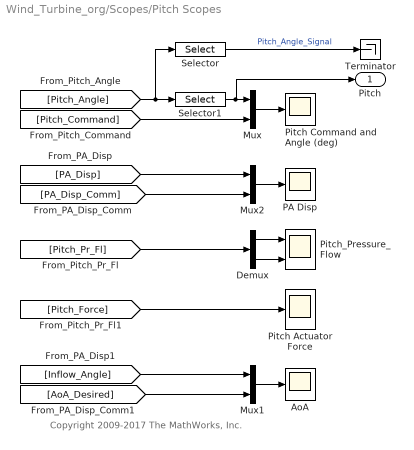
== system Wind_Turbine_org/Scopes/Pitch Scopes ==
  note: Copyright 2009-2017 The MathWorks, Inc.
  AoA : Scope
  Demux : Demux  Outputs=[2 1]
  Mux : Mux  Inputs=2
  Mux1 : Mux  Inputs=2
  Mux2 : Mux  Inputs=2
  PA Disp : Scope
  Pitch Actuator Force : Scope
  Pitch Command and Angle (deg) : Scope
  Pitch_Pressure_Flow : Scope  NumInputPorts=2
  Selector : Selector  InputPortWidth=3  IndexOptions=Index vector (dialog)  Indices=[1 ]  OutputSizes=1
  Selector1 : Selector  InputPortWidth=3  IndexOptions=Index vector (dialog)  Indices=[1 ]  OutputSizes=1
  Terminator : Terminator
  Pitch : Outport
  wires:
  [Pitch_Force] -> Pitch Actuator Force/1
  Selector/1 -> Terminator/1  "Pitch_Angle_Signal"
  Demux/2 -> Pitch_Pressure_Flow/2
  Demux/1 -> Pitch_Pressure_Flow/1
  [Pitch_Pr_Fl] -> Demux/1
  [PA_Disp_Comm] -> Mux2/2
  Mux2/1 -> PA Disp/1
  [PA_Disp] -> Mux2/1
  Mux/1 -> Pitch Command and Angle (deg)/1
  [Pitch_Command] -> Mux/2
  [Pitch_Angle] -> Selector/1, Selector1/1
  [AoA_Desired] -> Mux1/2
  Mux1/1 -> AoA/1
  [Inflow_Angle] -> Mux1/1
  Selector1/1 -> Pitch/1, Mux/1

== system Wind_Turbine_org/Scopes/Vis Off ==

== system Wind_Turbine_org/Scopes/Vis On ==

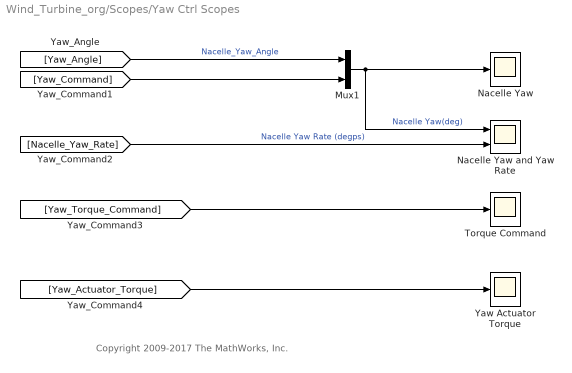
== system Wind_Turbine_org/Scopes/Yaw Ctrl Scopes ==
  note: Copyright 2009-2017 The MathWorks, Inc.
  Mux1 : Mux  Inputs=2
  Nacelle Yaw : Scope
  Nacelle Yaw and Yaw Rate : Scope  NumInputPorts=2
  Torque Command : Scope
  Yaw Actuator Torque : Scope
  wires:
  [Nacelle_Yaw_Rate] -> Nacelle Yaw and Yaw Rate/2  "Nacelle Yaw Rate (degps)"
  Mux1/1 -> Nacelle Yaw/1, Nacelle Yaw and Yaw Rate/1  "Nacelle Yaw(deg)"
  [Yaw_Command] -> Mux1/2
  [Yaw_Angle] -> Mux1/1  "Nacelle_Yaw_Angle"
  [Yaw_Torque_Command] -> Torque Command/1
  [Yaw_Actuator_Torque] -> Yaw Actuator Torque/1

== system Wind_Turbine_org/Scopes/tictoc1 ==

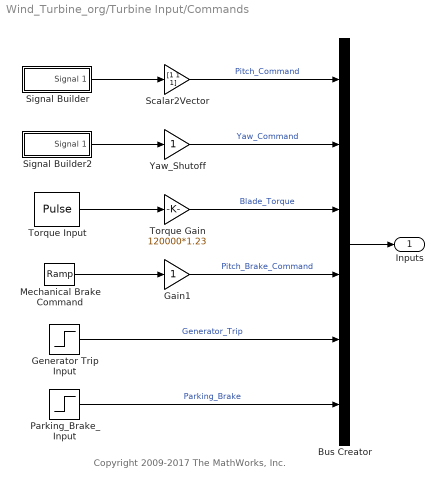
== system Wind_Turbine_org/Turbine Input/Commands ==
  note: Copyright 2009-2017 The MathWorks, Inc.
  Bus Creator : BusCreator  Inputs=6
  Gain1 : Gain
  Generator Trip Input : Step  Time=90  Before=1  SampleTime=0
  Mechanical Brake Command : simulink/Sources/Ramp  slope=1  start=40  InitialOutput=0
  Parking_Brake_Input : Step  Time=5  Before=1  After=0  SampleTime=0
  Scalar2Vector : Gain  Gain=[1 1 1]
  Signal Builder : Subsystem  Tag=STV Subsys  LoadFcn=sigbuilder_block('load');  StartFcn=sigbuilder_block('start');  StopFcn=sigbuilder_block('stop');  ClipboardFcn=sigbuilder_block('clipboard');  mask(Sigbuilder block){tuvar=[0:10]}
      mask help: Sigbuilder GUI
      mask init:
      | if ~strcmp(get_param(bdroot(gcbh),'SimulationStatus'),'stopped') tuvar = sigbuilder_block('maskInit'); end
      settings: CopyFcn=sigbuilder_block('copy');  DeleteFcn=sigbuilder_block('delete');  ModelCloseFcn=sigbuilder_block('modelClose');  PreSaveFcn=sigbuilder_block('preSave');  PauseFcn=sigbuilder_block('pause')  ContinueFcn=sigbuilder_block('continue')  NameChangeFcn=sigbuilder_block('namechange');  OpenFcn=sigbuilder_block('open',[214.5 254.25 550.5 399.75 ]);  CloseFcn=sigbuilder_block('close');
      mask Display: plot(0, 0, 100, 100,[2, 2, 32, 32, 2], [68, 8, 8, 68, 68],[32, 2], [38, 38], [32, 19, 2],[53, 60, 44], [32, 17, 17, 2],[16, 16, 31, 31]);txt = getActiveGroup(gcbh);text(2, 100, txt,'verticalAlignment', 'top');
  Signal Builder2 : Subsystem  Tag=STV Subsys  LoadFcn=sigbuilder_block('load');  StartFcn=sigbuilder_block('start');  StopFcn=sigbuilder_block('stop');  ClipboardFcn=sigbuilder_block('clipboard');  mask(Sigbuilder block){tuvar=[0:10]}
      mask help: Sigbuilder GUI
      mask init:
      | if ~strcmp(get_param(bdroot(gcbh),'SimulationStatus'),'stopped') tuvar = sigbuilder_block('maskInit'); end
      settings: CopyFcn=sigbuilder_block('copy');  DeleteFcn=sigbuilder_block('delete');  ModelCloseFcn=sigbuilder_block('modelClose');  PreSaveFcn=sigbuilder_block('preSave');  PauseFcn=sigbuilder_block('pause')  ContinueFcn=sigbuilder_block('continue')  NameChangeFcn=sigbuilder_block('namechange');  OpenFcn=sigbuilder_block('open',[28.5 161.25 550.5 489 ]);  CloseFcn=sigbuilder_block('close');
      mask Display: plot(0, 0, 100, 100,[2, 2, 32, 32, 2], [68, 8, 8, 68, 68],[32, 2], [38, 38], [32, 19, 2],[53, 60, 44], [32, 17, 17, 2],[16, 16, 31, 31]);txt = getActiveGroup(gcbh);text(2, 100, txt,'verticalAlignment', 'top');
  Torque Gain : Gain  Gain=120000*1.23
  Torque Input : DiscretePulseGenerator  PulseType=Time based  Amplitude=10  Period=100  PulseWidth=10
  Yaw_Shutoff : Gain
  Inputs : Outport
  wires:
  Bus Creator/1 -> Inputs/1
  Signal Builder2/1(Signal 1) -> Yaw_Shutoff/1
  Signal Builder/1(Signal 1) -> Scalar2Vector/1
  Torque Input/1 -> Torque Gain/1
  Scalar2Vector/1 -> Bus Creator/1  "Pitch_Command"
  Yaw_Shutoff/1 -> Bus Creator/2  "Yaw_Command"
  Torque Gain/1 -> Bus Creator/3  "Blade_Torque"
  Mechanical Brake Command/1 -> Gain1/1
  Generator Trip Input/1 -> Bus Creator/5  "Generator_Trip"
  Gain1/1 -> Bus Creator/4  "Pitch_Brake_Command"
  Parking_Brake_Input/1 -> Bus Creator/6  "Parking_Brake"

== system Wind_Turbine_org/Turbine Input/Wind ==
  Mux1 : Mux  Inputs=2
  Wind Input : Subsystem  Tag=STV Subsys  LoadFcn=sigbuilder_block('load');  StartFcn=sigbuilder_block('start');  StopFcn=sigbuilder_block('stop');  ClipboardFcn=sigbuilder_block('clipboard');  mask(Sigbuilder block){tuvar=[0:10]}
      mask help: Sigbuilder GUI
      mask init:
      | if ~strcmp(get_param(bdroot(gcbh),'SimulationStatus'),'stopped') tuvar = sigbuilder_block('maskInit'); end
      settings: CopyFcn=sigbuilder_block('copy');  DeleteFcn=sigbuilder_block('delete');  ModelCloseFcn=sigbuilder_block('modelClose');  PreSaveFcn=sigbuilder_block('preSave');  PauseFcn=sigbuilder_block('pause')  ContinueFcn=sigbuilder_block('continue')  NameChangeFcn=sigbuilder_block('namechange');  OpenFcn=sigbuilder_block('open',[17.4 220.2 762 360.6 ]);  CloseFcn=sigbuilder_block('close');
      mask Display: plot(0, 0, 100, 100,[2, 2, 32, 32, 2], [68, 8, 8, 68, 68],[32, 2], [38, 38], [32, 19, 2],[53, 60, 44], [32, 17, 17, 2],[16, 16, 31, 31]);txt = getActiveGroup(gcbh);text(2, 100, txt,'verticalAlignment', 'top');
  Inputs : Outport
  wires:
  Mux1/1 -> Inputs/1
  Wind Input/1(Wind Speed) -> Mux1/1
  Wind Input/2(Wind Direction) -> Mux1/2

== system Wind_Turbine_org/Scopes/Configure Turbine/Subsystem ==

== system Wind_Turbine_org/Scopes/Configure Turbine/Subsystem1 ==

== system Wind_Turbine_org/Scopes/Configure Turbine/Subsystem10 ==

== system Wind_Turbine_org/Scopes/Configure Turbine/Subsystem11 ==

== system Wind_Turbine_org/Scopes/Configure Turbine/Subsystem12 ==

== system Wind_Turbine_org/Scopes/Configure Turbine/Subsystem13 ==

== system Wind_Turbine_org/Scopes/Configure Turbine/Subsystem14 ==

== system Wind_Turbine_org/Scopes/Configure Turbine/Subsystem15 ==

== system Wind_Turbine_org/Scopes/Configure Turbine/Subsystem16 ==

== system Wind_Turbine_org/Scopes/Configure Turbine/Subsystem17 ==

== system Wind_Turbine_org/Scopes/Configure Turbine/Subsystem18 ==

== system Wind_Turbine_org/Scopes/Configure Turbine/Subsystem19 ==

== system Wind_Turbine_org/Scopes/Configure Turbine/Subsystem2 ==

== system Wind_Turbine_org/Scopes/Configure Turbine/Subsystem20 ==

== system Wind_Turbine_org/Scopes/Configure Turbine/Subsystem21 ==

== system Wind_Turbine_org/Scopes/Configure Turbine/Subsystem22 ==

== system Wind_Turbine_org/Scopes/Configure Turbine/Subsystem23 ==

== system Wind_Turbine_org/Scopes/Configure Turbine/Subsystem24 ==

== system Wind_Turbine_org/Scopes/Configure Turbine/Subsystem3 ==

== system Wind_Turbine_org/Scopes/Configure Turbine/Subsystem4 ==

== system Wind_Turbine_org/Scopes/Configure Turbine/Subsystem5 ==

== system Wind_Turbine_org/Scopes/Configure Turbine/Subsystem6 ==

== system Wind_Turbine_org/Scopes/Configure Turbine/Subsystem7 ==

== system Wind_Turbine_org/Scopes/Configure Turbine/Subsystem8 ==

== system Wind_Turbine_org/Scopes/Configure Turbine/Subsystem9 ==

== system Wind_Turbine_org/Turbine Input/Commands/Signal Builder ==
  Demux : Demux  Tag=STV Demux  Outputs=1
  FromWs : FromWorkspace  Tag=STV FromWs  VariableName=tuvar  SampleTime=0  SigBuilderData=DataTag0  VnvData=DataTag1
      SigBuilderData=|
      | common.afterFinalStr = 'Extrapolate'
      | common.sampleTime = 0
      | dataSet(1).timeRange = [0 50]
      | dataSet(1).name = 'Pos_Test'
      | dataSet(2).timeRange = [0 50]
      | dataSet(2).name = 'Pos_Neg_Test'
      | dataSet(3).timeRange = [0 50]
      | dataSet(3).name = 'Step_Test'
      | sbobj.Groups(1).Name = 'Pos_Test'
      | sbobj.Groups(1).Signals.Name = 'Signal 1'
      | sbobj.Groups(1).Signals.XData = [0 5 5 7.5 7.5 25.1 25.1 28 28 50]
      | sbobj.Groups(1).Signals.YData = [0 0 20 20 0 0 20 20 0 0]
      | sbobj.Groups(1).TimeRange = [0 50]
      | sbobj.Groups(2).Name = 'Pos_Neg_Test'
      | sbobj.Groups(2).Signals.Name = 'Signal 1'
      | sbobj.Groups(2).Signals.XData = [0 3 3 5.5 5.5 8 8 10.5 10.5 50]
      | sbobj.Groups(2).Signals.YData = [0 0 20 20 0 0 -20 -20 0 0]
      | sbobj.Groups(2).TimeRange = [0 50]
      | sbobj.Groups(3).Name = 'Step_Test'
      | sbobj.Groups(3).Signals.Name = 'Signal 1'
      | sbobj.Groups(3).Signals.XData = [0 1 1 7.5 25.1 30 30 50]
      | sbobj.Groups(3).Signals.YData = [0 0 20 20 20 20 0 0]
      | sbobj.Groups(3).TimeRange = [0 50]
  Signal 1 : Outport  Tag=STV Outport
  wires:
  Demux/1 -> Signal 1/1
  FromWs/1 -> Demux/1

== system Wind_Turbine_org/Turbine Input/Commands/Signal Builder2 ==
  Demux : Demux  Tag=STV Demux  Outputs=1
  FromWs : FromWorkspace  Tag=STV FromWs  VariableName=tuvar  SampleTime=0  SigBuilderData=DataTag2  VnvData=DataTag3
      SigBuilderData=|
      | common.afterFinalStr = 'Extrapolate'
      | common.sampleTime = 0
      | dataSet(1).timeRange = [0 50]
      | dataSet(1).name = 'Pos_Neg_Test'
      | dataSet(2).timeRange = [0 50]
      | dataSet(2).name = 'Step_Test'
      | dataSet(3).timeRange = [0 50]
      | dataSet(3).name = 'Ramp_Test'
      | sbobj.Groups(1).Name = 'Pos_Neg_Test'
      | sbobj.Groups(1).Signals.Name = 'Signal 1'
      | sbobj.Groups(1).Signals.XData = [0 1 1 11 11 21 21 31 31 50]
      | sbobj.Groups(1).Signals.YData = [0 0 4 4 0 0 -4 -4 0 0]
      | sbobj.Groups(2).Name = 'Step_Test'
      | sbobj.Groups(2).Signals.Name = 'Signal 1'
      | sbobj.Groups(2).Signals.XData = [0 1 1 11 21 31 31 50]
      | sbobj.Groups(2).Signals.YData = [0 0 4 4 4 4 0 0]
      | sbobj.Groups(3).Name = 'Ramp_Test'
      | sbobj.Groups(3).Signals.Name = 'Signal 1'
      | sbobj.Groups(3).Signals.XData = [0 1 1 11 21 31 39.1 50]
      | sbobj.Groups(3).Signals.YData = [0 0 2.46 4 2.32 3.18 1.16 0]
  Signal 1 : Outport  Tag=STV Outport
  wires:
  Demux/1 -> Signal 1/1
  FromWs/1 -> Demux/1

== system Wind_Turbine_org/Turbine Input/Wind/Wind Input ==
  Demux : Demux  Tag=STV Demux  Outputs=2
  FromWs : FromWorkspace  Tag=STV FromWs  VariableName=tuvar  SampleTime=0  SigBuilderData=DataTag4  VnvData=DataTag5
      SigBuilderData=|
      | common.afterFinalStr = 'Extrapolate'
      | common.sampleTime = 0
      | dataSet(1).timeRange = [0 130]
      | dataSet(1).name = 'Constant Wind No Yaw'
      | dataSet(2).timeRange = [0 130]
      | dataSet(2).name = 'Constant Wind'
      | dataSet(3).timeRange = [0 60]
      | dataSet(3).name = 'High Wind Speed'
      | dataSet(4).timeRange = [0 130]
      | dataSet(4).name = 'Cut Out'
      | dataSet(5).timeRange = [0 130]
      | dataSet(5).name = 'Start Stop'
      | dataSet(6).timeRange = [0 130]
      | dataSet(6).name = 'Start Stop No Yaw'
      | dataSet(7).timeRange = [0 130]
      | dataSet(7).name = 'Varying Wind'
      | sbobj.Groups(1).Name = 'Constant Wind No Yaw'
      | sbobj.Groups(1).Signals(1).Name = 'Wind Speed'
      | sbobj.Groups(1).Signals(1).XData = [0 10 130]
      | sbobj.Groups(1).Signals(1).YData = [10 10 10]
      | sbobj.Groups(1).Signals(2).Name = 'Wind Direction'
      | sbobj.Groups(1).Signals(2).XData = [0 1 11 21 31 130]
      | sbobj.Groups(1).Signals(2).YData = [0 0 0 0 0 0]
      | sbobj.Groups(2).Name = 'Constant Wind'
      | sbobj.Groups(2).Signals(1).Name = 'Wind Speed'
      | sbobj.Groups(2).Signals(1).XData = [0 10 130]
      | sbobj.Groups(2).Signals(1).YData = [10 10 10]
      | sbobj.Groups(2).Signals(2).Name = 'Wind Direction'
      | sbobj.Groups(2).Signals(2).XData = [0 1 1 11 11 21 21 31 31 130]
      | sbobj.Groups(2).Signals(2).YData = [0 0 4 4 0 0 -4 -4 0 0]
      | sbobj.Groups(3).Name = 'High Wind Speed'
      | sbobj.Groups(3).Signals(1).Name = 'Wind Speed'
      | sbobj.Groups(3).Signals(1).XData = [0 10 60]
      | sbobj.Groups(3).Signals(1).YData = [10 9.9 25]
      | sbobj.Groups(3).Signals(2).Name = 'Wind Direction'
      | sbobj.Groups(3).Signals(2).XData = [0 1 11 21 31 60]
      | sbobj.Groups(3).Signals(2).YData = [0 0 4 0 -2.1 0]
      | sbobj.Groups(4).Name = 'Cut Out'
      | sbobj.Groups(4).Signals(1).Name = 'Wind Speed'
      | sbobj.Groups(4).Signals(1).XData = [0 5 25.1 28 60 75 121.8 130]
      | sbobj.Groups(4).Signals(1).YData = [10 10 8.7 7.85 9.65 2 2 2]
      | sbobj.Groups(4).Signals(2).Name = 'Wind Direction'
      | sbobj.Groups(4).Signals(2).XData = [0 1 1 11 11 21 21 31 31 130]
      | sbobj.Groups(4).Signals(2).YData = [0 0 4 4 0 0 -4 -4 0 0]
      | sbobj.Groups(5).Name = 'Start Stop'
      | sbobj.Groups(5).Signals(1).Name = 'Wind Speed'
      | sbobj.Groups(5).Signals(1).XData = [0 5 25 28 55 75 80 130]
      | sbobj.Groups(5).Signals(1).YData = [2 2 13 10 15 2 2 2]
      | sbobj.Groups(5).Signals(2).Name = 'Wind Direction'
      | sbobj.Groups(5).Signals(2).XData = [0 1 11 21 31 36.6 54.8 75 130]
      | sbobj.Groups(5).Signals(2).YData = [0 0 2.9 0.5 0.5 1.57171717172 -4 -4 -4]
      | sbobj.Groups(6).Name = 'Start Stop No Yaw'
      | sbobj.Groups(6).Signals(1).Name = 'Wind Speed'
      | sbobj.Groups(6).Signals(1).XData = [0 5 25 28 55 75 80 130]
      | sbobj.Groups(6).Signals(1).YData = [2 2 13 10 15 2 2 2]
      | sbobj.Groups(6).Signals(2).Name = 'Wind Direction'
      | sbobj.Groups(6).Signals(2).XData = [0 130]
      | sbobj.Groups(6).Signals(2).YData = [0 0]
      | sbobj.Groups(7).Name = 'Varying Wind'
      | sbobj.Groups(7).Signals(1).Name = 'Wind Speed'
      | sbobj.Groups(7).Signals(1).XData = [0 5 25 28 45 60.2 75 78.2 80 130]
      | sbobj.Groups(7).Signals(1).YData = [2 2 13 10 14.4 10.6 13.9 8 8 2]
      | sbobj.Groups(7).Signals(2).Name = 'Wind Direction'
      | sbobj.Groups(7).Signals(2).XData = [0 1 11 21 31 36.6 54.8 75 130]
      | sbobj.Groups(7).Signals(2).YData = [0 0 2.9 0.5 0.5 1.57171717172 -4 -4 -4]
  Wind Speed : Outport  Tag=STV Outport
  Wind Direction : Outport  Tag=STV Outport  Port=2
  wires:
  Demux/2 -> Wind Direction/1
  Demux/1 -> Wind Speed/1
  FromWs/1 -> Demux/1
